simulink model "Simulink_model_Assignment"  (R2020b)
settings: Solver=VariableStepAuto  StartTime=0.0  StopTime=Time  RelTol=1e-3
values from neighbouring files (symbols this model uses):
  g = 9.81    [Integrated_EV_BMWi3_Script_Final.m]
  Grade = 0    [Integrated_EV_BMWi3_Script_Final.m]
  rho = 1.2    [Integrated_EV_BMWi3_Script_Final.m]
  WOT = 1    [Integrated_EV_BMWi3_Script_Final.m]
undefined symbols (not defined in the file or in its folder): Battery, Brake, DCDC, Motor, PID, vehicle
libraries: simulink x1
settings Model: Creator=hp  LastModifiedBy=adhip
settings DataIOCC: ExternalInput=[simtime, cyc_mps]  LoadExternalInput=on
settings SFSimCC: CustomCodeUndefinedFunction=UseInterfaceOnly

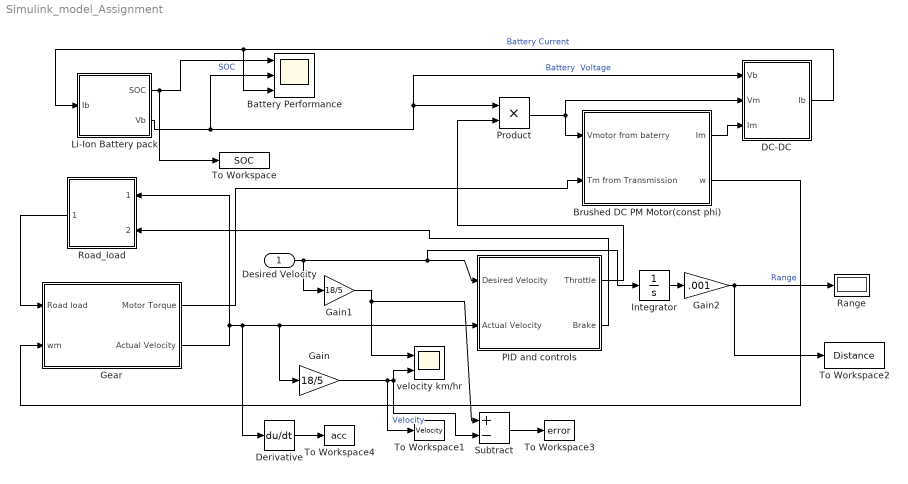
== system Simulink_model_Assignment ==
  Desired Velocity : Inport
  Battery Performance : Scope  NumInputPorts=3
  Brushed DC PM Motor(const phi) : Subsystem
  DC-DC : Subsystem
  Derivative : Derivative
  Gain : Gain  Gain=18/5
  Gain1 : Gain  Gain=18/5
  Gain2 : Gain  Gain=.001
  Gear : Subsystem
  Integrator : Integrator
  Li-Ion Battery pack : Subsystem
  PID and controls : Subsystem
  Product : Product
  Range : Display
  Road_load : Subsystem
  Subtract : Sum  Inputs=+-
  To Workspace : ToWorkspace  VariableName=SOC  SampleTime=1
  To Workspace1 : ToWorkspace  VariableName=Velocity  SampleTime=-1
  To Workspace2 : ToWorkspace  VariableName=Distance  SampleTime=1
  To Workspace3 : ToWorkspace  VariableName=error  SampleTime=1
  To Workspace4 : ToWorkspace  VariableName=acc  SampleTime=1
  velocity km/hr : Scope  NumInputPorts=2
  wires:
  Li-Ion Battery pack/1(SOC) -> To Workspace/1, Battery Performance/1  "SOC"
  Li-Ion Battery pack/2(Vb) -> Battery Performance/2, DC-DC/1(Vb), Product/1  "Battery  Voltage"
  Road_load/1(Road Load) -> Gear/1(Road load)
  Brushed DC PM Motor(const phi)/2(w) -> Gear/2(wm)
  Gear/1(Motor Torque) -> Brushed DC PM Motor(const phi)/2(Tm from Transmission)
  Product/1 -> DC-DC/2(Vm), Brushed DC PM Motor(const phi)/1(Vmotor from baterry)
  Brushed DC PM Motor(const phi)/1(Im) -> DC-DC/3(Im)
  DC-DC/1(Ib) -> Li-Ion Battery pack/1(Ib), Battery Performance/3  "Battery Current"
  Gain/1 -> To Workspace1/1, Subtract/2, velocity km/hr/2  "Velocity"
  PID and controls/2("Brake ") -> Road_load/2(Brake Signal)
  PID and controls/1(Throttle) -> Product/2
  Gear/2(Actual Velocity) -> Derivative/1, PID and controls/2(Actual Velocity), Gain/1, Road_load/1(velocity)
  Desired Velocity/1 -> Gain1/1, Integrator/1, PID and controls/1(Desired Velocity)
  Integrator/1 -> Gain2/1
  Gain2/1 -> Range/1, To Workspace2/1  "Range"
  Gain1/1 -> Subtract/1, velocity km/hr/1
  Subtract/1 -> To Workspace3/1
  Derivative/1 -> To Workspace4/1

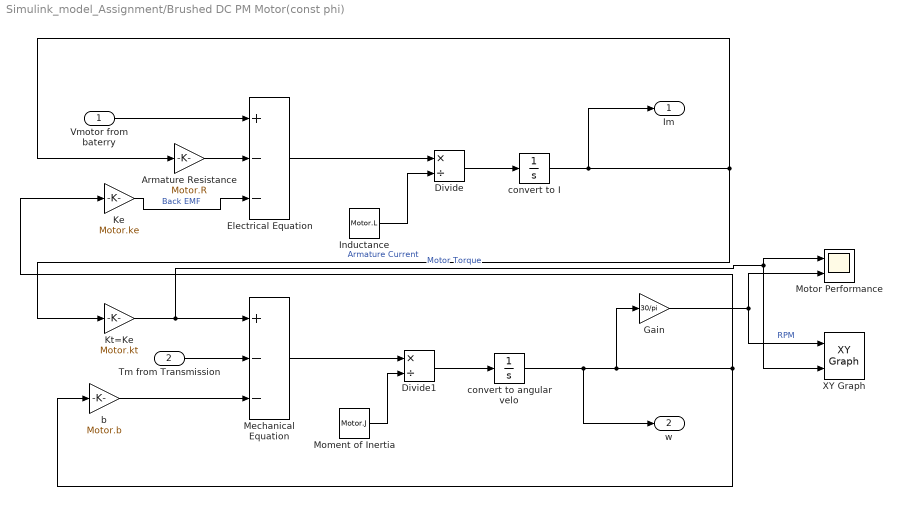
== system Simulink_model_Assignment/Brushed DC PM Motor(const phi) ==
  Vmotor from baterry : Inport
  Tm from Transmission : Inport  Port=2
  Armature Resistance : Gain  Gain=Motor.R
  Divide : Product  Inputs=*/
  Divide1 : Product  Inputs=*/
  Electrical Equation : Sum  Inputs=+--
  Gain : Gain  Gain=30/pi
  Inductance : Constant  Value=Motor.L
  Ke : Gain  Gain=Motor.ke
  Kt=Ke : Gain  Gain=Motor.kt
  Mechanical Equation : Sum  Inputs=+--
  Moment of Inertia : Constant  Value=Motor.J
  Motor Performance : Scope  NumInputPorts=2
  XY Graph : simulink/Sinks/XY Graph  xmin=0  xmax=12000  ymin=0  ymax=265  st=-1
  b : Gain  Gain=Motor.b
  convert to angular velo : Integrator
  "convert to I " : Integrator
  Im : Outport  VectorParamsAs1DForOutWhenUnconnected=off
  w : Outport  Port=2  VectorParamsAs1DForOutWhenUnconnected=off
  wires:
  Ke/1 -> Electrical Equation/3  "Back EMF"
  Divide/1 -> "convert to I "/1
  Armature Resistance/1 -> Electrical Equation/2
  Electrical Equation/1 -> Divide/1
  Inductance/1 -> Divide/2
  Mechanical Equation/1 -> Divide1/1
  "convert to I "/1 -> Armature Resistance/1, Kt=Ke/1, Im/1  "Armature Current"
  Kt=Ke/1 -> XY Graph/2, Motor Performance/1, Mechanical Equation/1  "Motor Torque"
  convert to angular velo/1 -> Ke/1, b/1, Gain/1, w/1
  b/1 -> Mechanical Equation/3
  Moment of Inertia/1 -> Divide1/2
  Tm from Transmission/1 -> Mechanical Equation/2
  Divide1/1 -> convert to angular velo/1
  Vmotor from baterry/1 -> Electrical Equation/1
  Gain/1 -> XY Graph/1, Motor Performance/2  "RPM"

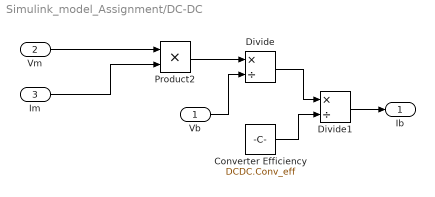
== system Simulink_model_Assignment/DC-DC ==
  Vb : Inport
  Vm : Inport  Port=2
  Im : Inport  Port=3
  Converter Efficiency : Constant  Value=DCDC.Conv_eff
  Divide : Product  Inputs=*/
  Divide1 : Product  Inputs=*/
  Product2 : Product
  Ib : Outport  VectorParamsAs1DForOutWhenUnconnected=off
  wires:
  Vb/1 -> Divide/2
  Product2/1 -> Divide/1
  Divide/1 -> Divide1/1
  Im/1 -> Product2/2
  Vm/1 -> Product2/1
  Converter Efficiency/1 -> Divide1/2
  Divide1/1 -> Ib/1

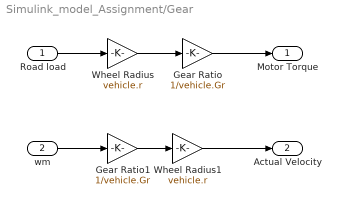
== system Simulink_model_Assignment/Gear ==
  Road load : Inport
  wm : Inport  Port=2
  Gear Ratio : Gain  Gain=1/vehicle.Gr
  Gear Ratio1 : Gain  Gain=1/vehicle.Gr
  Wheel Radius : Gain  Gain=vehicle.r
  Wheel Radius1 : Gain  Gain=vehicle.r
  Motor Torque : Outport  VectorParamsAs1DForOutWhenUnconnected=off
  Actual Velocity : Outport  Port=2  VectorParamsAs1DForOutWhenUnconnected=off
  wires:
  Road load/1 -> Wheel Radius/1
  wm/1 -> Gear Ratio1/1
  Wheel Radius/1 -> Gear Ratio/1
  Gear Ratio/1 -> Motor Torque/1
  Gear Ratio1/1 -> Wheel Radius1/1
  Wheel Radius1/1 -> Actual Velocity/1

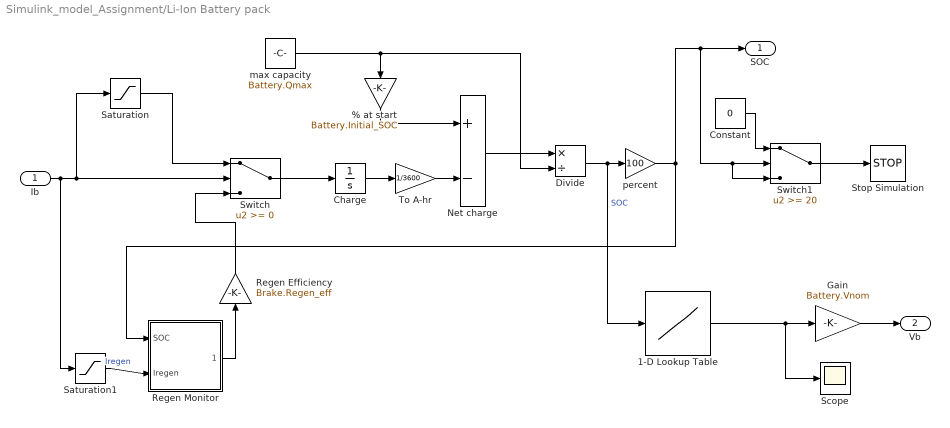
== system Simulink_model_Assignment/Li-Ion Battery pack ==
  Ib : Inport
  % at start : Gain  Gain=Battery.Initial_SOC
  1-D Lookup Table : Lookup_n-D  NumberOfTableDimensions=1  BreakpointsForDimension1=Battery.SOC  Table=Battery.normalized_voltage  InternalRulePriority=Speed  RndMeth=Simplest  InputSameDT=on
  Charge : Integrator
  Constant : Constant  Value=0
  Divide : Product  Inputs=*/
  Gain : Gain  Gain=Battery.Vnom
  Net charge : Sum  Inputs=+-
  Regen Efficiency : Gain  Gain=Brake.Regen_eff
  Regen Monitor : Subsystem
  Saturation : Saturate  UpperLimit=inf  LowerLimit=0
  Saturation1 : Saturate  UpperLimit=0  LowerLimit=-inf
  Scope : Scope
  Stop Simulation : Stop
  Switch : Switch
  Switch1 : Switch  Threshold=20
  To A-hr : Gain  Gain=1/3600
  max capacity : Constant  Value=Battery.Qmax
  percent : Gain  Gain=100
  SOC : Outport  VectorParamsAs1DForOutWhenUnconnected=off
  Vb : Outport  Port=2  VectorParamsAs1DForOutWhenUnconnected=off
  wires:
  Ib/1 -> Saturation/1, Switch/2, Saturation1/1
  Saturation/1 -> Switch/1
  Switch/1 -> Charge/1
  max capacity/1 -> Divide/2, % at start/1
  % at start/1 -> Net charge/1
  Charge/1 -> To A-hr/1
  Net charge/1 -> Divide/1
  Divide/1 -> 1-D Lookup Table/1, percent/1  "SOC"
  1-D Lookup Table/1 -> Scope/1, Gain/1
  percent/1 -> Regen Monitor/1(SOC), SOC/1, Switch1/3, Switch1/2
  Regen Monitor/1(Iregen allowed) -> Regen Efficiency/1
  Gain/1 -> Vb/1
  Regen Efficiency/1 -> Switch/3
  Saturation1/1 -> Regen Monitor/2(Iregen)  "Iregen"
  To A-hr/1 -> Net charge/2
  Switch1/1 -> Stop Simulation/1
  Constant/1 -> Switch1/1

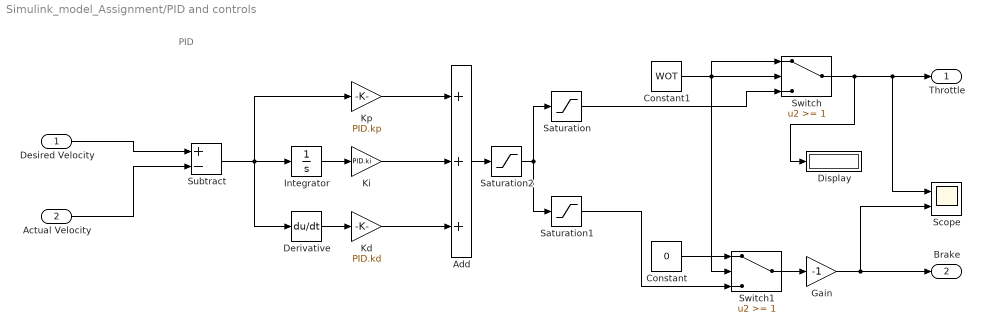
== system Simulink_model_Assignment/PID and controls ==
  note: PID
  Desired Velocity : Inport
  Actual Velocity : Inport  Port=2
  Add : Sum  Inputs=+++
  Constant : Constant  Value=0
  Constant1 : Constant  Value=WOT
  Derivative : Derivative
  Display : Display
  Gain : Gain  Gain=-1
  Integrator : Integrator
  Kd : Gain  Gain=PID.kd
  Ki : Gain  Gain=PID.ki
  Kp : Gain  Gain=PID.kp
  Saturation : Saturate  UpperLimit=1  LowerLimit=0
  Saturation1 : Saturate  UpperLimit=0  LowerLimit=-1
  Saturation2 : Saturate  UpperLimit=1  LowerLimit=-1
  Scope : Scope  NumInputPorts=2
  Subtract : Sum  Inputs=+-
  Switch : Switch  Threshold=1
  Switch1 : Switch  Threshold=1
  Throttle : Outport  VectorParamsAs1DForOutWhenUnconnected=off
  "Brake " : Outport  Port=2  VectorParamsAs1DForOutWhenUnconnected=off
  wires:
  Saturation/1 -> Switch/3
  Saturation1/1 -> Switch1/3
  Constant/1 -> Switch1/1
  Constant1/1 -> Switch1/2, Switch/1, Switch/2
  Switch1/1 -> Gain/1
  Subtract/1 -> Derivative/1, Kp/1, Integrator/1
  Actual Velocity/1 -> Subtract/2
  Desired Velocity/1 -> Subtract/1
  Ki/1 -> Add/2
  Derivative/1 -> Kd/1
  Integrator/1 -> Ki/1
  Kd/1 -> Add/3
  Add/1 -> Saturation2/1
  Kp/1 -> Add/1
  Switch/1 -> Scope/1, Throttle/1, Display/1
  Saturation2/1 -> Saturation1/1, Saturation/1
  Gain/1 -> "Brake "/1, Scope/2

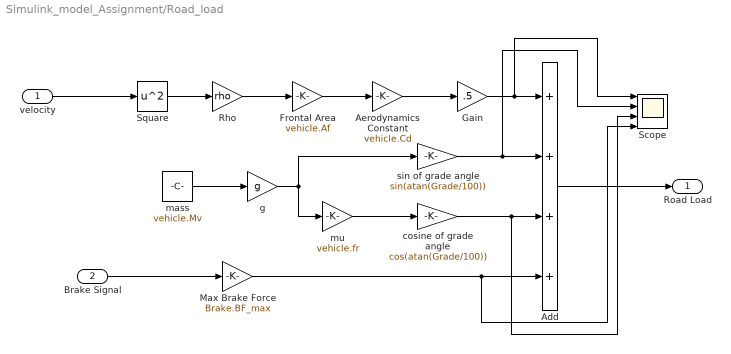
== system Simulink_model_Assignment/Road_load ==
  velocity : Inport
  Brake Signal : Inport  Port=2
  Add : Sum  Inputs=++++
  Aerodynamics Constant : Gain  Gain=vehicle.Cd
  Frontal Area : Gain  Gain=vehicle.Af
  Gain : Gain  Gain=.5
  Max Brake Force : Gain  Gain=Brake.BF_max
  Rho : Gain  Gain=rho
  Scope : Scope  NumInputPorts=4
  Square : Math  Operator=square  SignedPower=on  SaturateOnIntegerOverflow=on
  cosine of grade angle : Gain  Gain=cos(atan(Grade/100))
  g : Gain  Gain=g
  mass : Constant  Value=vehicle.Mv
  mu : Gain  Gain=vehicle.fr
  sin of grade angle : Gain  Gain=sin(atan(Grade/100))
  Road Load : Outport  VectorParamsAs1DForOutWhenUnconnected=off
  wires:
  velocity/1 -> Square/1
  Aerodynamics Constant/1 -> Gain/1
  Brake Signal/1 -> Max Brake Force/1
  cosine of grade angle/1 -> Scope/3, Add/3
  Gain/1 -> Scope/1, Add/1
  g/1 -> sin of grade angle/1, mu/1
  sin of grade angle/1 -> Scope/2, Add/2
  Add/1 -> Road Load/1
  Square/1 -> Rho/1
  Frontal Area/1 -> Aerodynamics Constant/1
  Rho/1 -> Frontal Area/1
  mass/1 -> g/1
  mu/1 -> cosine of grade angle/1
  Max Brake Force/1 -> Scope/4, Add/4

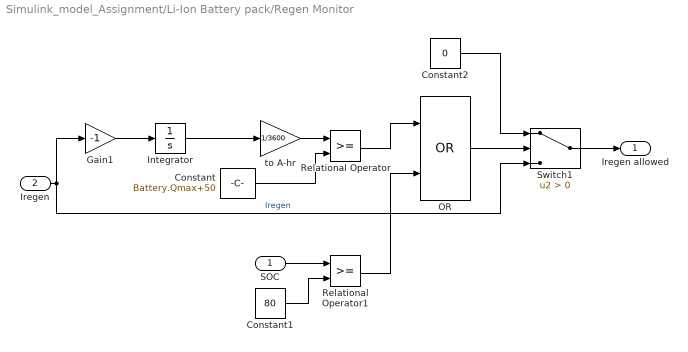
== system Simulink_model_Assignment/Li-Ion Battery pack/Regen Monitor ==
  SOC : Inport
  Iregen : Inport  Port=2
  Constant : Constant  Value=Battery.Qmax+50
  Constant1 : Constant  Value=80
  Constant2 : Constant  Value=0
  Gain1 : Gain  Gain=-1
  Integrator : Integrator
  OR : Logic  Operator=OR  IconShape=distinctive  AllPortsSameDT=off  OutDataTypeStr=boolean
  Relational Operator : RelationalOperator  OutDataTypeStr=boolean  RndMeth=Simplest
  Relational Operator1 : RelationalOperator  OutDataTypeStr=boolean  RndMeth=Simplest
  Switch1 : Switch  Criteria=u2 > Threshold
  to A-hr : Gain  Gain=1/3600
  Iregen allowed : Outport  VectorParamsAs1DForOutWhenUnconnected=off
  wires:
  Integrator/1 -> to A-hr/1
  Iregen/1 -> Gain1/1, Switch1/3  "Iregen"
  Relational Operator1/1 -> OR/2
  Constant1/1 -> Relational Operator1/2
  OR/1 -> Switch1/2
  Constant2/1 -> Switch1/1
  Relational Operator/1 -> OR/1
  to A-hr/1 -> Relational Operator/1
  Constant/1 -> Relational Operator/2
  Switch1/1 -> Iregen allowed/1
  SOC/1 -> Relational Operator1/1
  Gain1/1 -> Integrator/1
